simulink model "open_loop"  (R2018b)
settings: Solver=FixedStepAuto  StartTime=0.0  StopTime=10.0  FixedStep=1/100  MaxStep=1e-3  MinStep=1e-4  RelTol=1e-3  AbsTol=1e-3
model workspace: external: MATLAB File params.m (data not in the file)
values from neighbouring files (symbols this model uses):
  b = 2.75e-11    [Linearization_2.m]    (also in Linearizing.m; Linearizing_old.m; params.m)
  g = 9.81    [Linearization_2.m]    (also in Linearizing.m; Linearizing_old.m; params.m)
  k = 1e-9    (= 1e-09)    [Linearization_2.m]    (also in Linearizing.m; Linearizing_old.m; params.m)
  m = 0.027    [Linearization_2.m]    (also in Linearizing.m; Linearizing_old.m; params.m)
libraries: nesl_utility x9
settings Model: Creator=Jocke  LastModifiedBy=karst
settings SolverCC: AutoScaleAbsTol=off
settings SFSimCC: SimUseLocalCustomCode=off
settings RTWCC: RTWUseLocalCustomCode=off
settings CodeAppCC: StateflowObjectComments=on
settings SimscapeCC: SimscapeNormalizeSystem=off  SimscapeLogType=all  SimscapeLogLimitData=off  SimscapeLogDataHistory=10000

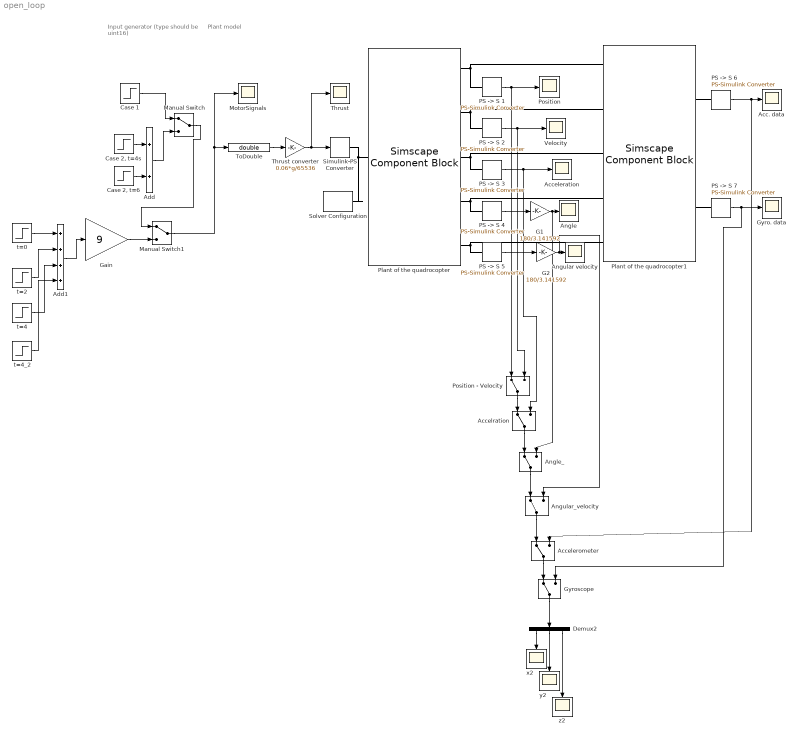
== system open_loop ==
  note: Input generator
      | (type should be uint16)
  note: Plant model
  Acc. data : Scope
  Acceleration : Scope
  Accelerometer : ManualSwitch
  Accelration : ManualSwitch
  Add : Sum
  Add1 : Sum  Inputs=++++
  Angle : Scope
  Angle_ : ManualSwitch
  Angular velocity : Scope
  Angular_velocity : ManualSwitch
  Case 1 : Step  Time=4  Before=[0;0;0;0]  After=[10;10;0;0]  SampleTime=0
  "Case 2, t=4s" : Step  Time=4  Before=[0;0;0;0]  After=[1000;0;0;0]  SampleTime=0
  "Case 2, t=6" : Step  Time=6  Before=[0;0;0;0]  After=[0;0;2000;0]  SampleTime=0
  Demux2 : Demux  Outputs=3
  G1 : Gain  Gain=180/3.141592
  G2 : Gain  Gain=180/3.141592
  Gain : Gain  Gain=9
  Gyro. data : Scope
  Gyroscope : ManualSwitch
  Manual Switch : ManualSwitch
  Manual Switch1 : ManualSwitch
  MotorSignals : Scope
  PS -> S {1..7} (7 alike) : nesl_utility/PS-Simulink Converter  PhysicalDomain=network_engine_domain  SubClassName=ps_output  LeftPortType=input  RightPortType=output  PseudoPeriodic=off  Frequencies=[]  Unit=1  AffineConversion=off
  Plant of the quadrocopter : SimscapeComponentBlock  SourceFile=plant  ComponentPath=plant  ComponentVariants=plant  ComponentVariantNames=plant  ClassName=plant  SchemaVersion=1  m=m kg  g=g m/s^2  d=d m  k=k  b=b
      settings: CopyFcn=simscape.engine.sli.internal.componentblockcallback(gcbh,'COPY')  PreCopyFcn=simscape.engine.sli.internal.componentblockcallback(gcbh,'PRECOPY')  PreDeleteFcn=simscape.engine.sli.internal.componentblockcallback(gcbh,'PREDELETE')
      mask Type: Plant of quadrocopter
  Plant of the quadrocopter1 : SimscapeComponentBlock  SourceFile=sensors  ComponentPath=sensors  ComponentVariants=sensors  ComponentVariantNames=sensors  ClassName=sensors  SchemaVersion=1  m=m kg  g=g m/s^2  d=d m  k=k  b=b
      settings: CopyFcn=simscape.engine.sli.internal.componentblockcallback(gcbh,'COPY')  PreCopyFcn=simscape.engine.sli.internal.componentblockcallback(gcbh,'PRECOPY')  PreDeleteFcn=simscape.engine.sli.internal.componentblockcallback(gcbh,'PREDELETE')
      mask Type: Plant of quadrocopter
  Position : Scope
  Position - Velocity : ManualSwitch
  Simulink-PS Converter : nesl_utility/Simulink-PS Converter  PhysicalDomain=network_engine_domain  SubClassName=ps_input  LeftPortType=input  RightPortType=output  PseudoPeriodic=off  Frequencies=[]  NoiseDistribution=none  NoiseParameters=[]  Unit=1  AffineConversion=off  FilteringAndDerivatives=zero  SimscapeFilterOrder=1  InputFilterTimeConstant=0.001  UdotUserProvided=1
  Solver Configuration : nesl_utility/Solver Configuration  PhysicalDomain=network_engine_domain  SubClassName=solver  LeftPortType=input  RightPortType=generic  Tones=[]  Harmonics=[]  SimulateNoise=off  Profile=off  UseLocalSampling=off  EnableSwitchedLinearOptims=on  FrequencyDomain=off  UseCCode=off  RelTol=0.001  AbsTol=1e-06  MinStep=1e-09  ToWorkspace=off  RevertToSquareIcSolve=off  NumHomotopyIterations=100  PhasorMode=off  PhasorModeNumHarmonics=1  DoDC=off  ResidualTolerance=1e-09  UseLocalSolver=off  LocalSolverChoice=NE_BACKWARD_EULER_ADVANCER  LocalSolverSampleTime=0.001  DoFixedCost=off  MaxNonlinIter=3  MaxModeIter=2  LinearAlgebra=Sparse  EquationFormulation=NE_TIME_EF  DelaysMemoryBudget=1024  AutomaticFiltering=on  FilteringTimeConstant=0.001  PartitionStorageMethod=AS_NEEDED  PartitionMemoryBudget=1024
  Thrust : Scope
  Thrust converter : Gain  Gain=0.06*g/65536
  ToDouble : DataTypeConversion  OutDataTypeStr=double  RndMeth=Round  SaturateOnIntegerOverflow=on
  Velocity : Scope
  t=0 : Step  Time=0  Before=[0;0;0;0]  After=[1;0;0;1]  SampleTime=0
  t=2 : Step  Time=2  Before=[0;0;0;0]  After=[-1;1;1;-1]  SampleTime=0
  t=4 : Step  Time=4  Before=[0;0;0;0]  After=[0;-1;-1;0]  SampleTime=0
  t=4_2 : Step  Time=4  Before=[0;0;0;0]  After=[10;10;10;10]  SampleTime=0
  x2 : Scope
  y2 : Scope
  z2 : Scope
  wires:
  "PS -> S 7"/1 -> Gyro. data/1, Gyroscope/2
  "PS -> S 6"/1 -> Accelerometer/2, Acc. data/1
  G1/1 -> Angle_/2, Angle/1
  G2/1 -> Angular_velocity/2, Angular velocity/1
  ToDouble/1 -> Thrust converter/1
  Thrust converter/1 -> Thrust/1, Simulink-PS Converter/1
  "PS -> S 1"/1 -> Position - Velocity/1, Position/1
  "PS -> S 5"/1 -> G2/1
  "PS -> S 4"/1 -> G1/1
  "PS -> S 3"/1 -> Accelration/2, Acceleration/1
  "PS -> S 2"/1 -> Position - Velocity/2, Velocity/1
  Case 1/1 -> Manual Switch/1
  "Case 2, t=4s"/1 -> Add/1
  "Case 2, t=6"/1 -> Add/2
  Add/1 -> Manual Switch/2
  Position - Velocity/1 -> Accelration/1
  Angle_/1 -> Angular_velocity/1
  Accelration/1 -> Angle_/1
  Demux2/2 -> y2/1
  Demux2/1 -> x2/1
  Gyroscope/1 -> Demux2/1
  Demux2/3 -> z2/1
  Angular_velocity/1 -> Accelerometer/1
  Accelerometer/1 -> Gyroscope/1
  Manual Switch1/1 -> MotorSignals/1, ToDouble/1
  Manual Switch/1 -> Manual Switch1/1
  Gain/1 -> Manual Switch1/2
  t=0/1 -> Add1/1
  t=2/1 -> Add1/2
  t=4/1 -> Add1/3
  Add1/1 -> Gain/1
  t=4_2/1 -> Add1/4
  connections:
  Plant of the quadrocopter/LConn1 -- Simulink-PS Converter/RConn1 -- Solver Configuration/RConn1
  Plant of the quadrocopter/RConn1 -- Plant of the quadrocopter1/LConn1 -- "PS -> S 1"/LConn1
  Plant of the quadrocopter/RConn2 -- Plant of the quadrocopter1/LConn2 -- "PS -> S 2"/LConn1
  Plant of the quadrocopter/RConn3 -- Plant of the quadrocopter1/LConn3 -- "PS -> S 3"/LConn1
  Plant of the quadrocopter/RConn4 -- Plant of the quadrocopter1/LConn4 -- "PS -> S 4"/LConn1
  Plant of the quadrocopter/RConn5 -- Plant of the quadrocopter1/LConn5 -- "PS -> S 5"/LConn1
  Plant of the quadrocopter1/RConn1 -- "PS -> S 6"/LConn1
  Plant of the quadrocopter1/RConn2 -- "PS -> S 7"/LConn1
